simulink model "sldemo_adc_quantize"  (R2024a)
settings: Solver=VariableStepDiscrete  StartTime=0.0  StopTime=6000  FixedStep=0.1  MaxStep=0.1  RelTol=1e-3  EnableMultiTasking=on
StartFcn:
  | if exist('adc_ploth')
  |   if ishghandle(adc_ploth,'figure')
  |     close(adc_ploth)
  |   end
  |   clear adc_ploth
  | end
StopFcn:
  | if exist('yout')
  |  if isstruct(yout)
  |   adc_ploth = figure;
  |   plot(yout.signals(1).values,double(yout.signals(2).values),'bo-'), grid, hold on, plot([0,4096],[0,4096],'g'), hold off
  |   title(sprintf('Idealized A/D converter quantization algorithm \n (Zoom in close with the mouse to see behavior details)'))
  |   zoom on
  |  end
  | end
libraries: simulink_extras x1, simulink x1
CloseFcn:
  | if exist('adc_ploth')
  |   if ishghandle(adc_ploth,'figure')
  |     close(adc_ploth)
  |   end
  |   clear adc_ploth
  |   if exist('tout'), clear tout; end
  |   if exist('yout'), clear yout; end
  | end
Description:
  | Analog-to-Digital Converter Quantization Algorithm
  | 
  | The quantization algorithm in the model takes in a 0 to 5 volt signal and outputs
  | a 12-bit digital word in a 16-bit signed integer. A value of 0 corresponds to 0 Volts
  | and a value of 4096 would correspond to 5 Volts. A change in the least
  | significant bit (LSB) is about 1.2 mV. As 12 bits can only reach the value of
  | 4095, the highest voltage that can be read by this device is approximately
  | 4.9988 Volts. In order to have no more than 1/2 LSB error, the quantizer changes
  | values midway between each voltage point, resulting in a 1/2-width interval at
  | 0 Volts and a 3/2-width interval just below 5 Volts.
settings Model: Creator=The MathWorks, Inc.  LastModifiedBy=neham
settings SolverCC: AlgebraicLoopSolver=TrustRegion
settings DataIOCC: ExternalInput=ustruct  MaxDataPoints=5000  SaveFormat=StructureWithTime  ReturnWorkspaceOutputs=off
settings OptimizationCC: BooleanDataType=off  DefaultParameterBehavior=Inlined  InlineInvariantSignals=on  ExpressionDepthLimit=2147483647  ZeroExternalMemoryAtStartup=off  InitFltsAndDblsToZero=on  LifeSpan=1  BufferReusableBoundary=off  EfficientTunableParamExpr=on
settings DebuggingCC: SaveWithParameterizedLinksMsg=none  UnderspecifiedInitializationDetection=Classic  MergeDetectMultiDrivingBlocksExec=none  CheckExecutionContextPreStartOutputMsg=on  SignalResolutionControl=TryResolveAllWithWarning  SolverPrmCheckMsg=warning  MultiTaskDSMMsg=warning  MultiTaskCondExecSysMsg=none  FcnCallInpInsideContextMsg=warning  UnconnectedInputMsg=warning  UnconnectedOutputMsg=warning  UnconnectedLineMsg=warning  BusObjectLabelMismatch=none  StateNameClashWarn=warning  SFUnexpectedBacktrackingDiag=warning  SFNoUnconditionalDefaultTransitionDiag=warning  SFExecutionAtInitializationDiag=none  ArithmeticOperatorsInVariantConditions=warning
settings HardwareCC: ProdBitPerPointer=32  ProdBitPerSizeT=32  ProdBitPerPtrDiffT=32  ProdLargestAtomicFloat=None  ProdIntDivRoundTo=Undefined  ProdEndianess=Unspecified  ProdWordSize=32  ProdHWDeviceType=32-bit Generic
settings ModelReferenceCC: EnableRefExpFcnMdlSchedulingChecks=on  PropagateSignalLabelsOutOfModel=off
settings SFSimCC: SimUseLocalCustomCode=off  SimParseCustomCode=off  CustomCodeUndefinedFunction=UseInterfaceOnly
settings RTWCC: Description=RTW Embedded Coder (no auto configuration)  SystemTargetFile=ert.tlc  TemplateMakefile=ert_default_tmf  RTWUseLocalCustomCode=off  GPUComputeCapability=3.5
settings CodeAppCC: CustomSymbolStrType=$N$R$M  CustomSymbolStrFcn=$F$N$M  DefineNamingRule=UpperCase  StateflowObjectComments=on  InternalIdentifier=Classic  InlinedPrmAccess=Macros
settings ERTTargetCC: TargetFcnLib=iso_tfl_tmw.mat  TargetLangStandard=C99 (ISO)  UtilityFuncGeneration=Shared location  MultiwordLength=2048  GenerateSampleERTMain=on  SuppressErrorStatus=on  SupportAbsoluteTime=off  SupportNonFinite=off  SupportComplex=off  InlinedParameterPlacement=NonHierarchical  ERTCustomFileTemplate=example_file_process.tlc  ConvertIfToSwitch=off  SuppressUnreachableDefaultCases=off
settings ConfigComp: CovMetricSettings=dw  CovSaveCumulativeToWorkspaceVar=on  CovSaveSingleToWorkspaceVar=on  CovExternalEMLEnable=off

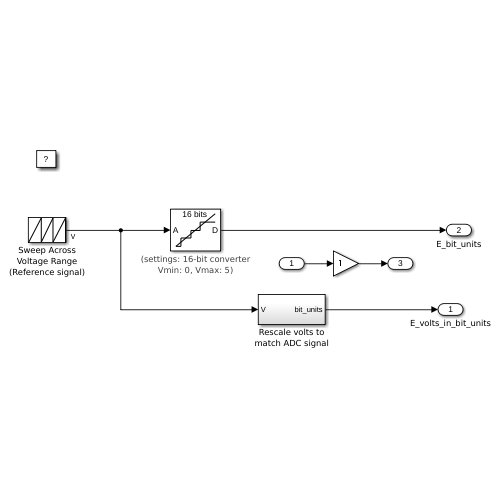
[thumbnail: Simulink's stored preview of the top-level diagram]
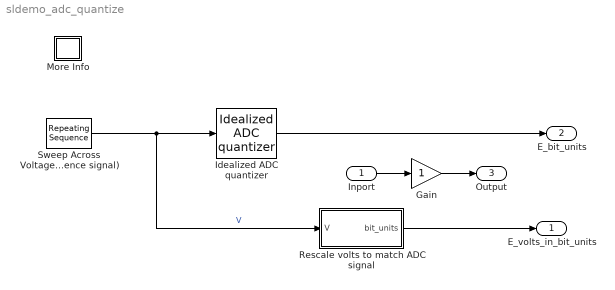
== system sldemo_adc_quantize ==
  Inport : Inport
  Gain : Gain
  Idealized ADC quantizer : simulink_extras/Additional Discrete/Idealized ADC quantizer  NumberOfConverterBits=16  Vmin=0  Vmax=5  OutputDataType=int16  OutputNegativeValues=off
  More Info : Subsystem
      settings: OpenFcn=showExample('simulink_general/sldemo_tc_scriptExample')
      mask Display: disp('?')
  Rescale volts to match ADC signal : Subsystem
  Sweep Across Voltage Range (Reference signal) : simulink/Sources/Repeating Sequence  rep_seq_t=[0 700]  rep_seq_y=[-0.25, 7]
  E_volts_in_bit_units : Outport  VectorParamsAs1DForOutWhenUnconnected=off
  E_bit_units : Outport  Port=2  VectorParamsAs1DForOutWhenUnconnected=off
  Output : Outport  Port=3
  wires:
  Sweep Across Voltage Range (Reference signal)/1 -> Rescale volts to match ADC signal/1(V), Idealized ADC quantizer/1  "V"
  Idealized ADC quantizer/1 -> E_bit_units/1
  Rescale volts to match ADC signal/1(bit_units) -> E_volts_in_bit_units/1
  Inport/1 -> Gain/1
  Gain/1 -> Output/1

== system sldemo_adc_quantize/More Info ==

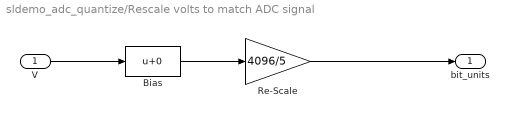
== system sldemo_adc_quantize/Rescale volts to match ADC signal ==
  V : Inport
  Bias : Bias  SaturateOnIntegerOverflow=off
  Re-Scale : Gain  Gain=4096/5
  bit_units : Outport  VectorParamsAs1DForOutWhenUnconnected=off
  wires:
  Bias/1 -> Re-Scale/1
  V/1 -> Bias/1
  Re-Scale/1 -> bit_units/1
